simulink model "AdaptiveSuspensionSystem"  (R2024b)
settings: Solver=ode45  StartTime=0.0  StopTime=10.0  MaxStep=0.01  RelTol=1e-3
settings Model: Creator=Anirudh  LastModifiedBy=Anirudh

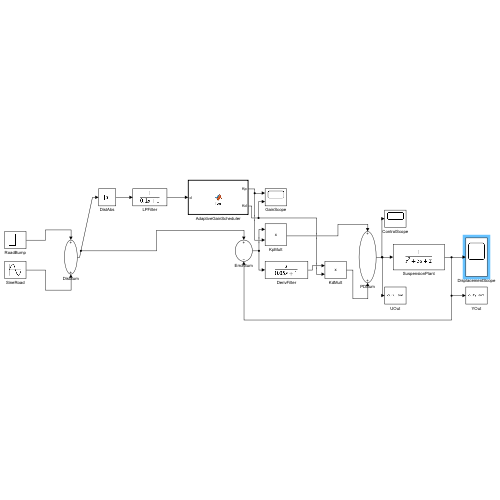
[thumbnail: Simulink's stored preview of the top-level diagram]
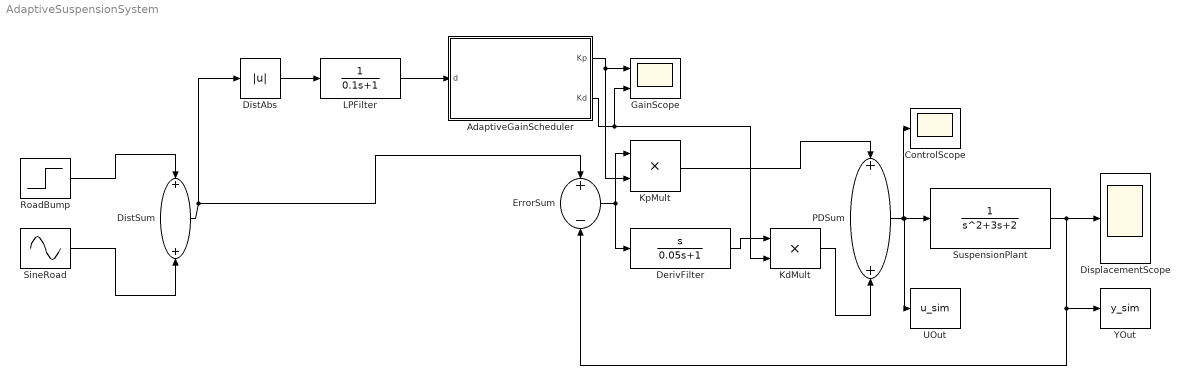
== system AdaptiveSuspensionSystem ==
  AdaptiveGainScheduler : MATLAB Function  TreatAsAtomicUnit=on
  ControlScope : Scope
  DerivFilter : TransferFcn  Numerator=[1, 0]  Denominator=[0.05, 1]
  DisplacementScope : Scope
  DistAbs : Abs  SaturateOnIntegerOverflow=off
  DistSum : Sum
  ErrorSum : Sum  Inputs=+-
  GainScope : Scope  NumInputPorts=2
  KdMult : Product
  KpMult : Product
  LPFilter : TransferFcn  Denominator=[0.1, 1]
  PDSum : Sum
  RoadBump : Step  Time=2  SampleTime=0
  SineRoad : Sin  Amplitude=0.01  Frequency=3.14159  SampleTime=0
  SuspensionPlant : TransferFcn  Denominator=[1, 3, 2]
  UOut : ToWorkspace  VariableName=u_sim  SaveFormat=Timeseries  SampleTime=-1
  YOut : ToWorkspace  VariableName=y_sim  SaveFormat=Timeseries  SampleTime=-1
  wires:
  DistSum/1 -> ErrorSum/1, DistAbs/1
  DistAbs/1 -> LPFilter/1
  LPFilter/1 -> AdaptiveGainScheduler/1(d)
  AdaptiveGainScheduler/1(Kp) -> KpMult/2, GainScope/1
  ErrorSum/1 -> DerivFilter/1, KpMult/1
  AdaptiveGainScheduler/2(Kd) -> GainScope/2, KdMult/2
  DerivFilter/1 -> KdMult/1
  KpMult/1 -> PDSum/1
  KdMult/1 -> PDSum/2
  PDSum/1 -> ControlScope/1, UOut/1, SuspensionPlant/1
  SuspensionPlant/1 -> YOut/1, ErrorSum/2, DisplacementScope/1
  RoadBump/1 -> DistSum/1
  SineRoad/1 -> DistSum/2

== matlab function AdaptiveSuspensionSystem/AdaptiveGainScheduler ==
  data: d input; Kp output; Kd output
function [Kp,Kd] = fcn(d)

Kp = 25 + 10*d;

Kd = 20 + 8*d;

end
